simulink model "model_pid"  (R2013a)
settings: Solver=ode45  StartTime=0.0  StopTime=10.0  RelTol=1e-3
values from neighbouring files (symbols this model uses):
  k1 = 10    [skrypt.m]
  k2 = 6    [skrypt.m]
  Td = 3    [lab4.m]    (also in skrypt.m = 5)
  Tp = 0.2    [skrypt.m]
  x = 0:pi/36:10*pi    [odp_sinus.m]    (also in skrypt.m = 0)
settings Model: Creator=L13-4  LastModifiedBy=Dawid Perdek
settings DataIOCC: SignalLoggingSaveFormat=ModelDataLogs
settings DebuggingCC: UnderspecifiedInitializationDetection=Simplified  MultiTaskDSMMsg=warning  MultiTaskCondExecSysMsg=none  StateNameClashWarn=none  StrictBusMsg=ErrorOnBusTreatedAsVector
settings RTWCC: IncludeERTFirstTime=on
settings GRTTargetCC: CodeReplacementLibrary=None  CPPClassGenCompliant=on

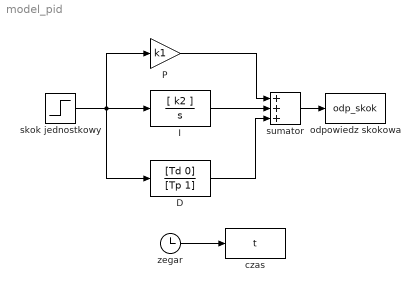
== system model_pid ==
  D : TransferFcn  Numerator=[Td 0]  Denominator=[Tp 1]
  I : TransferFcn  Numerator=[ k2 ]  Denominator=[1 0]
  P : Gain  Gain=k1
  czas : ToWorkspace  VariableName=t  SampleTime=-1
  odpowiedz skokowa : ToWorkspace  VariableName=odp_skok  SampleTime=-1
  skok jednostkowy : Step  Time=x  SampleTime=0
  sumator : Sum  Inputs=+++
  zegar : Clock
  wires:
  skok jednostkowy/1 -> I/1, D/1, P/1
  D/1 -> sumator/3
  P/1 -> sumator/1
  sumator/1 -> odpowiedz skokowa/1
  zegar/1 -> czas/1
  I/1 -> sumator/2
